simulink model "QPSK_Mod_demod"  (R2015a)
settings: Solver=ode45  StartTime=0.0  StopTime=12  RelTol=1e-3
libraries: powerlib_meascontrol x1
settings Model: Creator=user  LastModifiedBy=hp
settings DebuggingCC: UnderspecifiedInitializationDetection=Classic  MergeDetectMultiDrivingBlocksExec=none  SolverPrmCheckMsg=warning  StateNameClashWarn=warning

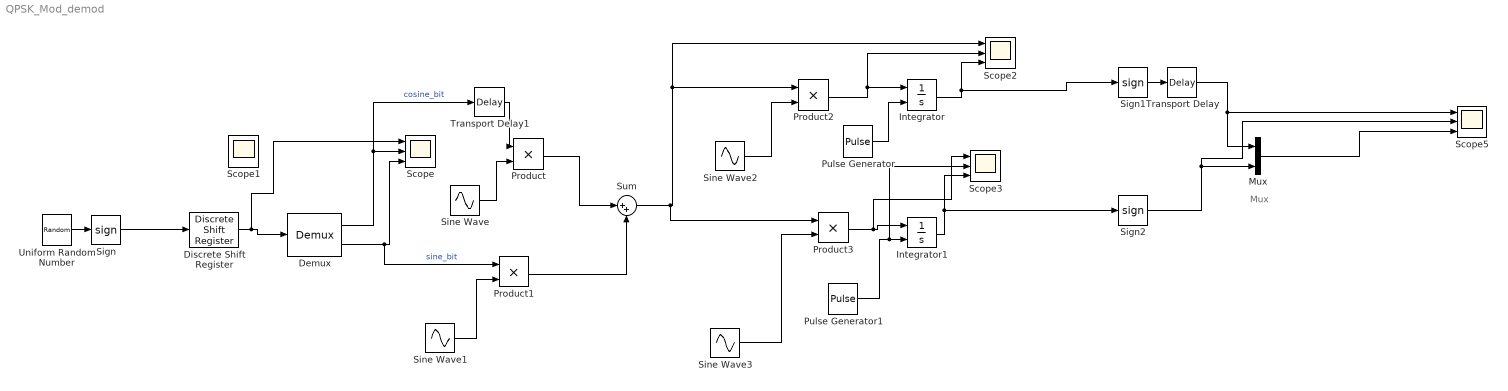
== system QPSK_Mod_demod ==
  note: Mux
  Demux : Demux  Outputs=2
  Discrete Shift Register : powerlib_meascontrol/Additional Components/Discrete Shift Register  NSamples=2  InitialValue=0  Ts=1
  Integrator : Integrator  ExternalReset=level  LimitOutput=on
  Integrator1 : Integrator  ExternalReset=level
  Mux : Mux  Inputs=2
  Product{,1..3} (4 alike) : Product
  Pulse Generator : DiscretePulseGenerator  PulseType=Time based  PhaseDelay=1
  Pulse Generator1 : DiscretePulseGenerator  PulseType=Time based  PhaseDelay=1
  Scope{,2..3,5} (4 alike) : Scope  NumInputPorts=3
      Scope settings: YMin=-5~-5~-5  YMax=5~5~5
      Scope2 settings: YMin=-5~-5~-5  YMax=5~5~5  SaveName=ScopeData2
      Scope3 settings: YMin=-5~-5~-5  YMax=5~5~5  SaveName=ScopeData3
      Scope5 settings: YMin=-5~-5~-5  YMax=5~5~5  SaveName=ScopeData5
  Scope1 : Scope
      settings: TimeRange=12  YMin=-1  YMax=1
  Sign : Signum
  Sign1 : Signum
  Sign2 : Signum
  Sine Wave : Sin  Frequency=2*pi*5  Phase=pi/2  SampleTime=.01
  Sine Wave1 : Sin  Frequency=2*pi*5  SampleTime=.01
  Sine Wave2 : Sin  Frequency=2*pi*5  Phase=pi/2  SampleTime=.01
  Sine Wave3 : Sin  Frequency=2*pi*5  SampleTime=.01
  Sum : Sum  Inputs=|++
  Transport Delay : TransportDelay
  Transport Delay1 : TransportDelay
  Uniform Random Number : UniformRandomNumber  SampleTime=1
  wires:
  Uniform Random Number/1 -> Sign/1
  Discrete Shift Register/1 -> Scope/1, Demux/1
  Demux/2 -> Product1/1, Scope/3  "sine_bit"
  Product/1 -> Sum/1
  Product1/1 -> Sum/2
  Sine Wave1/1 -> Product1/2
  Sine Wave/1 -> Product/2
  Demux/1 -> Transport Delay1/1, Scope/2  "cosine_bit"
  Sum/1 -> Product3/1, Scope2/1, Product2/1
  Sine Wave3/1 -> Product3/2
  Sine Wave2/1 -> Product2/2
  Product2/1 -> Scope2/2, Integrator/1
  Pulse Generator/1 -> Integrator/2
  Pulse Generator1/1 -> Scope3/2, Integrator1/2
  Product3/1 -> Scope3/1, Integrator1/1
  Integrator/1 -> Sign1/1, Scope2/3
  Integrator1/1 -> Sign2/1, Scope3/3
  Sign/1 -> Discrete Shift Register/1
  Transport Delay1/1 -> Product/1
  Sign1/1 -> Transport Delay/1
  Transport Delay/1 -> Scope5/1, Mux/1
  Sign2/1 -> Scope5/2, Mux/2
  Mux/1 -> Scope5/3
